simulink model "main"  (R2021a)
settings: Solver=ode45  StartTime=0.0  StopTime=200  RelTol=1e-3  EnableMultiTasking=on
libraries: spsDiodeLib x6, spsVoltageMeasurementLib x5, spsGroundLib x3, spsControlledVoltageSourceLib x3, spsSeriesRLCBranchLib x1, spspowerguiLib x1
settings Model: Creator=Waqas vicky  LastModifiedBy=ahm_e
settings SolverCC: AlgebraicLoopSolver=TrustRegion
settings DataIOCC: LimitDataPoints=on  SaveFormat=Array  SignalLoggingSaveFormat=ModelDataLogs  ReturnWorkspaceOutputs=off
settings OptimizationCC: ExpressionDepthLimit=2147483647  LifeSpan=inf
settings DebuggingCC: UnderspecifiedInitializationDetection=Classic  MergeDetectMultiDrivingBlocksExec=none  SolverPrmCheckMsg=warning  FcnCallInpInsideContextMsg=warning  StateNameClashWarn=warning  SFUnexpectedBacktrackingDiag=warning  SFNoUnconditionalDefaultTransitionDiag=warning  SFExecutionAtInitializationDiag=none  SFMachineParentedDataDiag=warning  ArithmeticOperatorsInVariantConditions=warning
settings HardwareCC: ProdBitPerPointer=32  ProdBitPerSizeT=32  ProdBitPerPtrDiffT=32  ProdLargestAtomicFloat=None  ProdIntDivRoundTo=Undefined  ProdEndianess=Unspecified  ProdWordSize=32  ProdHWDeviceType=32-bit Generic
settings ModelReferenceCC: PropagateSignalLabelsOutOfModel=off
settings SFSimCC: SimUseLocalCustomCode=off  CustomCodeUndefinedFunction=UseInterfaceOnly
settings RTWCC: RTWUseLocalCustomCode=off
settings CodeAppCC: StateflowObjectComments=on
settings GRTTargetCC: TargetLangStandard=C89/C90 (ANSI)  CombineOutputUpdateFcns=off  GRTInterface=on
settings ConfigComp: CovMetricSettings=dw  CovSaveCumulativeToWorkspaceVar=on  CovSaveSingleToWorkspaceVar=on  CovExternalEMLEnable=off
settings SimscapeCC: SimscapeNormalizeSystem=off

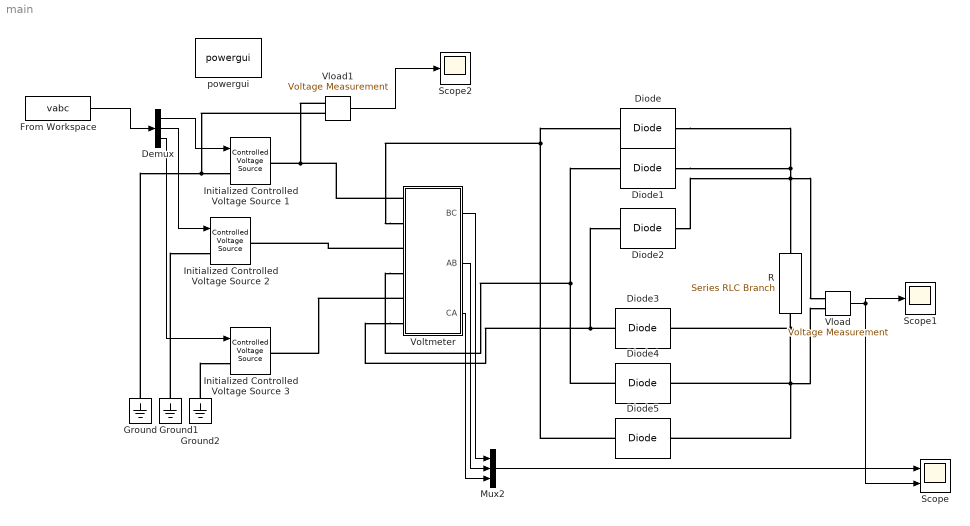
== system main ==
  Demux : Demux  Outputs=3
  Diode{,1..5} (6 alike) : spsDiodeLib/Diode  Ron=0.001  Lon=0  Vf=0.8  IC=0  UseSnubber=off  Rs=500  Cs=250e-9  Measurements=off
  From Workspace : FromWorkspace  VariableName=vabc
  Ground : spsGroundLib/Ground  LConnTagsString=a
  Ground1 : spsGroundLib/Ground  LConnTagsString=a
  Ground2 : spsGroundLib/Ground  LConnTagsString=a
  Initialized Controlled Voltage Source 1 : spsControlledVoltageSourceLib/Controlled Voltage Source  Description=source block  Initialize=on  Source_Type=AC  Amplitude=120  Phase=0  Frequency=60  Measurements=None
      settings: AttributesFormatString=\n
  Initialized Controlled Voltage Source 2 : spsControlledVoltageSourceLib/Controlled Voltage Source  Description=source block  Initialize=on  Source_Type=AC  Amplitude=120  Phase=0  Frequency=60  Measurements=None
      settings: AttributesFormatString=\n
  Initialized Controlled Voltage Source 3 : spsControlledVoltageSourceLib/Controlled Voltage Source  Description=source block  Initialize=on  Source_Type=AC  Amplitude=120  Phase=0  Frequency=60  Measurements=None
      settings: AttributesFormatString=\n
  Mux2 : Mux  Inputs=3
  R : spsSeriesRLCBranchLib/Series RLC Branch  LConnTagsString=__new0  RConnTagsString=__new0  BranchType=R  Resistance=1  Inductance=1e-3  SetiL0=off  InitialCurrent=0  Capacitance=1e-6  Setx0=off  InitialVoltage=0  Measurements=None
  Scope : Scope  NumInputPorts=2
  Scope1 : Scope
  Scope2 : Scope
  Vload : spsVoltageMeasurementLib/Voltage Measurement  PhasorSimulation=off  OutputType=Complex  PSBequivalent=0
  Vload1 : spsVoltageMeasurementLib/Voltage Measurement  PhasorSimulation=off  OutputType=Complex  PSBequivalent=0
  Voltmeter : Subsystem
  powergui : spspowerguiLib/powergui  Priority=1  SimulationMode=Continuous  SampleTime=50e-6  frequency=60  Iterations=50  frequencyindice=0  Pbase=100e6  ErrMax=1e-4  UnitsV=kV  UnitsW=MW  buscounter=0  FunctionMessages=off  echomessages=off  EnableUseOfTLC=off  CurrentSourceSwitches=on  DisableSnubberDevices=off  DisableRonSwitches=off  DisableVfSwitches=off  DisplayEquations=off  AutomaticDiscreteSolvers=off  SolverType=Tustin  Interpol=off  ExternalGateDelay=off  methode=off  Ts=100  x0status=blocks  SPID=off  SwTol=0  HookPort=off  NonlinearTolerance=1e-4  nMaxIteration=100  ContinueOnMaxIteration=off  RestoreLinks=warning  ResistiveCurrentMeasurement=off  Frange=[0:2:500]  Ylog=off  Xlog=on  ShowGrid=off  save=off  variable=ZData  structure=0  ZoomFFT=off  StartTime=0.0  cycles=1  DisplayStyle=1  fundamental=60  FreqAxis=off  MaxFrequency=1000  frequencyindicesteady=1  RmsSteady=1  display=off
  wires:
  Voltmeter/1(BC) -> Mux2/1
  Voltmeter/2(AB) -> Mux2/2
  Voltmeter/3(CA) -> Mux2/3
  Vload/1 -> Scope/2, Scope1/1
  Mux2/1 -> Scope/1
  Demux/1 -> Initialized Controlled Voltage Source 1/1
  Demux/2 -> Initialized Controlled Voltage Source 2/1
  Demux/3 -> Initialized Controlled Voltage Source 3/1
  Vload1/1 -> Scope2/1
  From Workspace/1 -> Demux/1
  connections:
  Voltmeter/LConn6 -- Diode2/LConn1 -- Diode3/RConn1
  Voltmeter/LConn4 -- Diode4/RConn1 -- Diode1/LConn1
  Voltmeter/LConn2 -- Diode5/RConn1 -- Diode/LConn1
  Ground/LConn1 -- Vload1/LConn2 -- Initialized Controlled Voltage Source 1/LConn1
  Ground1/LConn1 -- Initialized Controlled Voltage Source 2/LConn1
  Ground2/LConn1 -- Initialized Controlled Voltage Source 3/LConn1
  Diode2/RConn1 -- Diode/RConn1 -- Diode1/RConn1 -- Vload/LConn1 -- R/LConn1
  Vload/LConn2 -- Diode4/LConn1 -- Diode5/LConn1 -- Diode3/LConn1 -- R/RConn1
  Voltmeter/LConn1 -- Vload1/LConn1 -- Initialized Controlled Voltage Source 1/RConn1
  Voltmeter/LConn3 -- Initialized Controlled Voltage Source 2/RConn1
  Voltmeter/LConn5 -- Initialized Controlled Voltage Source 3/RConn1

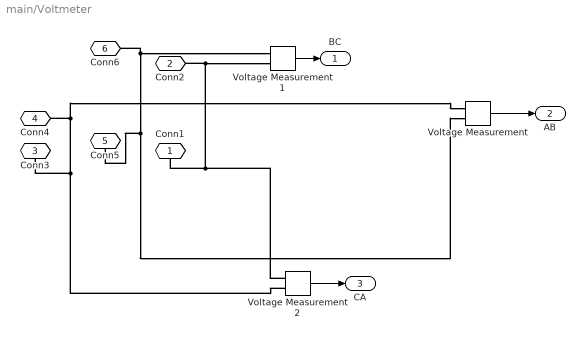
== system main/Voltmeter ==
  Voltage Measurement : spsVoltageMeasurementLib/Voltage Measurement  PhasorSimulation=off  OutputType=Complex  PSBequivalent=0
  Voltage Measurement1 : spsVoltageMeasurementLib/Voltage Measurement  PhasorSimulation=off  OutputType=Complex  PSBequivalent=0
  Voltage Measurement2 : spsVoltageMeasurementLib/Voltage Measurement  PhasorSimulation=off  OutputType=Complex  PSBequivalent=0
  Conn1 : PMIOPort  Side=Left
  Conn2 : PMIOPort  Port=2  Side=Left
  Conn3 : PMIOPort  Port=3  Side=Left
  Conn4 : PMIOPort  Port=4  Side=Left
  Conn5 : PMIOPort  Port=5  Side=Left
  Conn6 : PMIOPort  Port=6  Side=Left
  BC : Outport
  AB : Outport  Port=2
  CA : Outport  Port=3
  wires:
  Voltage Measurement1/1 -> BC/1
  Voltage Measurement/1 -> AB/1
  Voltage Measurement2/1 -> CA/1
  connections:
  Conn4/RConn1 -- Voltage Measurement/LConn1 -- Voltage Measurement2/LConn2 -- Conn3/RConn1
  Conn6/RConn1 -- Voltage Measurement1/LConn1 -- Voltage Measurement/LConn2 -- Conn5/RConn1
  Conn2/RConn1 -- Voltage Measurement1/LConn2 -- Voltage Measurement2/LConn1 -- Conn1/RConn1
